simulink model "StarkQuadSimCL7772"  (R2018b)
settings: Solver=ode15s  StartTime=0.0  StopTime=Final_Time_1  RelTol=1e-3
values from neighbouring files (symbols this model uses):
  b = 1.0444e-4    (= 0.00010444)    [StarkQuad77.m]
  d = 7.3031e-6    (= 7.3031e-06)    [StarkQuad77.m]
  g = 9.81    [StarkQuad77.m]
  Index = int32(Index)    [StarkQuad77.m]
  Ixx = 5.296671410    (= 5.29667141)    [StarkQuad77.m]
  Iyy = 5.790964671    [StarkQuad77.m]
  Izz = 3.348512883    [StarkQuad77.m]
  l = 0.41123*2    (= 0.82246)    [StarkQuad77.m]
  M = [x z y]    [StarkQuad77.m]
  m = 10.800    (= 10.8)    [StarkQuad77.m]
  Psi_d = 10    [StarkQuad77.m]
  u1_max = b*4*speed_rads^2    (= 106.539244)    [StarkQuad77.m]
  u1_min = 0    [StarkQuad77.m]
  u2_max = b*l*speed_rads^2    (= 21.9060666551)    [StarkQuad77.m]
  u2_min = -u2_max    (= -21.9060666551)    [StarkQuad77.m]
  u3_max = u2_max    (= 21.9060666551)    [StarkQuad77.m]
  u3_min = u2_min    (= -21.9060666551)    [StarkQuad77.m]
  u4_max = d*l*2*speed_rads^2    (= 3.06361921464)    [StarkQuad77.m]
  u4_min = -u4_max    (= -3.06361921464)    [StarkQuad77.m]
  xp = CP.x(end)    [StarkQuad77.m]
  yp = CP.y(end)    [StarkQuad77.m]
libraries: simulink x6, powerlib_meascontrol x3, aerolibutil x2, vrlib x1
settings Model: Creator=cindyiskandar  LastModifiedBy=Anthony

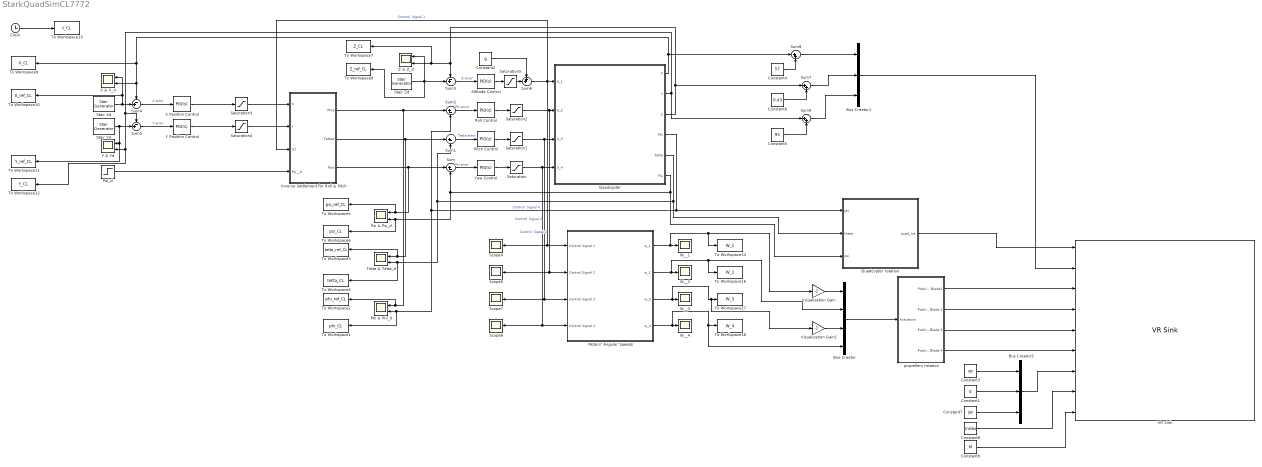
== system StarkQuadSimCL7772 ==
  "Altitude Control " : simulink/Continuous/PID Controller  Controller=PID  Form=Parallel  TimeDomain=Continuous-time  SampleTime=-1  IntegratorMethod=Forward Euler  FilterMethod=Forward Euler  ControllerParametersSource=internal  P=450  I=25  D=600  UseFilter=on  N=100  TunerSelectOption=Transfer Function Based (PID Tuner App)  InitialConditionSource=internal  InitialConditionForIntegrator=0  InitialConditionForFilter=0  DifferentiatorICPrevScaledInput=0  ExternalReset=none  TrackingMode=off  Kt=1  LimitOutput=off  UpperSaturationLimit=inf  LowerSaturationLimit=-inf  LinearizeAsGain=on  AntiWindupMode=none  Kb=1  POutMin=[]  POutMax=[]  IOutMin=[]  IOutMax=[]  DOutMin=[]  DOutMax=[]  NOutMin=[]  NOutMax=[]  SumOutMin=[]  SumOutMax=[]  SaturationOutMin=[]  SaturationOutMax=[]  PParamMin=[]  PParamMax=[]  IParamMin=[]  IParamMax=[]  DParamMin=[]  DParamMax=[]  NParamMin=[]  NParamMax=[]  KbParamMin=[]  KbParamMax=[]  KtParamMin=[]  KtParamMax=[]  KbOutMin=[]  KbOutMax=[]  KtOutMin=[]  KtOutMax=[]  IntegratorOutMin=[]  IntegratorOutMax=[]  FilterOutMin=[]  FilterOutMax=[]  SumI1OutMin=[]  SumI1OutMax=[]  SumI2OutMin=[]  SumI2OutMax=[]  SumI3OutMin=[]  SumI3OutMax=[]  SumI4OutMin=[]  SumI4OutMax=[]  SumDOutMin=[]  SumDOutMax=[]  DifferentiatorOutMin=[]  DifferentiatorOutMax=[]  FilterDiffOutCoefMin=[]  FilterDiffOutCoefMax=[]  ReciprocalOutMin=[]  ReciprocalOutMax=[]  SumDenOutMin=[]  SumDenOutMax=[]  SumNumOutMin=[]  SumNumOutMax=[]  DivideOutMin=[]  DivideOutMax=[]  IntegratorContinuousStateAttributes=''  IntegratorStateMustResolveToSignalObject=off  IntegratorRTWStateStorageClass=Auto  FilterContinuousStateAttributes=''  FilterStateMustResolveToSignalObject=off  FilterRTWStateStorageClass=Auto  ParallelPVariant=InternalParameters  IdealPVariant=Disabled  IVariant=InternalParameters  DVariant=InternalParameters  IntegratorVariant=Continuous  SatVariant=Disabled  AWVariant=Passthrough  PCopyVariant=Disabled  TRVariant=Disabled  FdbkBlocksVariant=Forward  IdealPFdbkVariant=Disabled  SatFdbkVariant=Disabled  DerivativeFilterVariant=ContFilter  NVariant=InternalParameters  NCopyVariant=Disabled  FilterICVariant=InternalICsFilter  IntegratorICVariant=InternalICs  ExternalResetVariant=Disabled  TRSumVariant=Passthrough  SumFdbkVariant=Disabled  SumVariant=Sum_PID
  Bus Creator : BusCreator  Inputs=4
  Bus Creator1 : BusCreator  Inputs=3
  Bus Creator2 : BusCreator  Inputs=3
  Clock : Clock
  Constant1 : Constant  Value=0
  Constant2 : Constant  Value=g
  Constant3 : Constant  Value=xp
  Constant4 : Constant  Value=57
  Constant5 : Constant  Value=95
  Constant6 : Constant  Value=0.43
  Constant7 : Constant  Value=yp
  Constant8 : Constant  Value=Index  VectorParams1D=off
  Constant9 : Constant  Value=M
  Inverse Settlement for Roll & Pitch : Subsystem
  Motors' Angular Speeds : Subsystem
  "Phi & Phi_d " : Scope  NumInputPorts=2
  Pitch Control : simulink/Continuous/PID Controller  Controller=PID  Form=Parallel  TimeDomain=Continuous-time  SampleTime=-1  IntegratorMethod=Forward Euler  FilterMethod=Forward Euler  ControllerParametersSource=internal  P=226  I=0  D=320  UseFilter=on  N=100  TunerSelectOption=Transfer Function Based (PID Tuner App)  InitialConditionSource=internal  InitialConditionForIntegrator=0  InitialConditionForFilter=0  DifferentiatorICPrevScaledInput=0  ExternalReset=none  TrackingMode=off  Kt=1  LimitOutput=off  UpperSaturationLimit=inf  LowerSaturationLimit=-inf  LinearizeAsGain=on  AntiWindupMode=none  Kb=1  POutMin=[]  POutMax=[]  IOutMin=[]  IOutMax=[]  DOutMin=[]  DOutMax=[]  NOutMin=[]  NOutMax=[]  SumOutMin=[]  SumOutMax=[]  SaturationOutMin=[]  SaturationOutMax=[]  PParamMin=[]  PParamMax=[]  IParamMin=[]  IParamMax=[]  DParamMin=[]  DParamMax=[]  NParamMin=[]  NParamMax=[]  KbParamMin=[]  KbParamMax=[]  KtParamMin=[]  KtParamMax=[]  KbOutMin=[]  KbOutMax=[]  KtOutMin=[]  KtOutMax=[]  IntegratorOutMin=[]  IntegratorOutMax=[]  FilterOutMin=[]  FilterOutMax=[]  SumI1OutMin=[]  SumI1OutMax=[]  SumI2OutMin=[]  SumI2OutMax=[]  SumI3OutMin=[]  SumI3OutMax=[]  SumI4OutMin=[]  SumI4OutMax=[]  SumDOutMin=[]  SumDOutMax=[]  DifferentiatorOutMin=[]  DifferentiatorOutMax=[]  FilterDiffOutCoefMin=[]  FilterDiffOutCoefMax=[]  ReciprocalOutMin=[]  ReciprocalOutMax=[]  SumDenOutMin=[]  SumDenOutMax=[]  SumNumOutMin=[]  SumNumOutMax=[]  DivideOutMin=[]  DivideOutMax=[]  IntegratorContinuousStateAttributes=''  IntegratorStateMustResolveToSignalObject=off  IntegratorRTWStateStorageClass=Auto  FilterContinuousStateAttributes=''  FilterStateMustResolveToSignalObject=off  FilterRTWStateStorageClass=Auto  ParallelPVariant=InternalParameters  IdealPVariant=Disabled  IVariant=InternalParameters  DVariant=InternalParameters  IntegratorVariant=Continuous  SatVariant=Disabled  AWVariant=Passthrough  PCopyVariant=Disabled  TRVariant=Disabled  FdbkBlocksVariant=Forward  IdealPFdbkVariant=Disabled  SatFdbkVariant=Disabled  DerivativeFilterVariant=ContFilter  NVariant=InternalParameters  NCopyVariant=Disabled  FilterICVariant=InternalICsFilter  IntegratorICVariant=InternalICs  ExternalResetVariant=Disabled  TRSumVariant=Passthrough  SumFdbkVariant=Disabled  SumVariant=Sum_PID
  Psi & Psi_d : Scope  NumInputPorts=2
  Psi_d : Step  After=Psi_d  SampleTime=0
  Quadcopter : Subsystem
  Quadcopter rotation : Subsystem
  Roll Control : simulink/Continuous/PID Controller  Controller=PID  Form=Parallel  TimeDomain=Continuous-time  SampleTime=-1  IntegratorMethod=Forward Euler  FilterMethod=Forward Euler  ControllerParametersSource=internal  P=290  I=0  D=320  UseFilter=on  N=100  TunerSelectOption=Transfer Function Based (PID Tuner App)  InitialConditionSource=internal  InitialConditionForIntegrator=0  InitialConditionForFilter=0  DifferentiatorICPrevScaledInput=0  ExternalReset=none  TrackingMode=off  Kt=1  LimitOutput=off  UpperSaturationLimit=inf  LowerSaturationLimit=-inf  LinearizeAsGain=on  AntiWindupMode=none  Kb=1  POutMin=[]  POutMax=[]  IOutMin=[]  IOutMax=[]  DOutMin=[]  DOutMax=[]  NOutMin=[]  NOutMax=[]  SumOutMin=[]  SumOutMax=[]  SaturationOutMin=[]  SaturationOutMax=[]  PParamMin=[]  PParamMax=[]  IParamMin=[]  IParamMax=[]  DParamMin=[]  DParamMax=[]  NParamMin=[]  NParamMax=[]  KbParamMin=[]  KbParamMax=[]  KtParamMin=[]  KtParamMax=[]  KbOutMin=[]  KbOutMax=[]  KtOutMin=[]  KtOutMax=[]  IntegratorOutMin=[]  IntegratorOutMax=[]  FilterOutMin=[]  FilterOutMax=[]  SumI1OutMin=[]  SumI1OutMax=[]  SumI2OutMin=[]  SumI2OutMax=[]  SumI3OutMin=[]  SumI3OutMax=[]  SumI4OutMin=[]  SumI4OutMax=[]  SumDOutMin=[]  SumDOutMax=[]  DifferentiatorOutMin=[]  DifferentiatorOutMax=[]  FilterDiffOutCoefMin=[]  FilterDiffOutCoefMax=[]  ReciprocalOutMin=[]  ReciprocalOutMax=[]  SumDenOutMin=[]  SumDenOutMax=[]  SumNumOutMin=[]  SumNumOutMax=[]  DivideOutMin=[]  DivideOutMax=[]  IntegratorContinuousStateAttributes=''  IntegratorStateMustResolveToSignalObject=off  IntegratorRTWStateStorageClass=Auto  FilterContinuousStateAttributes=''  FilterStateMustResolveToSignalObject=off  FilterRTWStateStorageClass=Auto  ParallelPVariant=InternalParameters  IdealPVariant=Disabled  IVariant=InternalParameters  DVariant=InternalParameters  IntegratorVariant=Continuous  SatVariant=Disabled  AWVariant=Passthrough  PCopyVariant=Disabled  TRVariant=Disabled  FdbkBlocksVariant=Forward  IdealPFdbkVariant=Disabled  SatFdbkVariant=Disabled  DerivativeFilterVariant=ContFilter  NVariant=InternalParameters  NCopyVariant=Disabled  FilterICVariant=InternalICsFilter  IntegratorICVariant=InternalICs  ExternalResetVariant=Disabled  TRSumVariant=Passthrough  SumFdbkVariant=Disabled  SumVariant=Sum_PID
  Saturation : Saturate  UpperLimit=u4_max  LowerLimit=u4_min
  Saturation1 : Saturate  UpperLimit=u3_max  LowerLimit=u3_min
  Saturation2 : Saturate  UpperLimit=u2_max  LowerLimit=u2_min
  Saturation3 : Saturate  UpperLimit=3*g  LowerLimit=-3*g
  Saturation4 : Saturate  UpperLimit=3*g  LowerLimit=-3*g
  Saturation5 : Saturate  UpperLimit=u1_max  LowerLimit=u1_min
  Scope{4..7} (4 alike) : Scope
  Stair Xd : powerlib_meascontrol/Pulse & Signal Generators/Stair Generator  t=Time  e=Xd  Ts=0
      settings: SourceProductName=Simscape Power Systems
  Stair Yd : powerlib_meascontrol/Pulse & Signal Generators/Stair Generator  t=Time  e=Yd  Ts=0
      settings: SourceProductName=Simscape Power Systems
  Stair Zd : powerlib_meascontrol/Pulse & Signal Generators/Stair Generator  t=Time  e=Zd  Ts=0
      settings: SourceProductName=Simscape Power Systems
  Sum : Sum  Inputs=|+-
  Sum1 : Sum  Inputs=|+-
  Sum2 : Sum  Inputs=|+-
  Sum3 : Sum  Inputs=-+|
  Sum4 : Sum  Inputs=-+|
  Sum5 : Sum  Inputs=-+|
  Sum6 : Sum  Inputs=++|
  Sum7 : Sum  Inputs=|++
  Sum8 : Sum  Inputs=|++
  Sum9 : Sum  Inputs=|++
  "Tetta & Tetta_d " : Scope  NumInputPorts=2
  To Workspace1 : ToWorkspace  VariableName=phi_CL  SampleTime=-1
      settings: Save2DSignal=2-D array (concatenate along first dimension)
  To Workspace10 : ToWorkspace  VariableName=X_ref_CL  SampleTime=-1
      settings: Save2DSignal=2-D array (concatenate along first dimension)
  To Workspace11 : ToWorkspace  VariableName=Y_ref_CL  SampleTime=-1
      settings: Save2DSignal=2-D array (concatenate along first dimension)
  To Workspace12 : ToWorkspace  VariableName=Y_CL  SampleTime=-1
      settings: Save2DSignal=2-D array (concatenate along first dimension)
  To Workspace13 : ToWorkspace  VariableName=t_CL  SampleTime=-1
      settings: Save2DSignal=2-D array (concatenate along first dimension)
  To Workspace14 : ToWorkspace  VariableName=W_1  SampleTime=-1
      settings: Save2DSignal=2-D array (concatenate along first dimension)
  To Workspace16 : ToWorkspace  VariableName=W_2  SampleTime=-1
      settings: Save2DSignal=2-D array (concatenate along first dimension)
  To Workspace17 : ToWorkspace  VariableName=W_3  SampleTime=-1
      settings: Save2DSignal=2-D array (concatenate along first dimension)
  To Workspace18 : ToWorkspace  VariableName=W_4  SampleTime=-1
      settings: Save2DSignal=2-D array (concatenate along first dimension)
  To Workspace2 : ToWorkspace  VariableName=phi_ref_CL  SampleTime=-1
      settings: Save2DSignal=2-D array (concatenate along first dimension)
  To Workspace3 : ToWorkspace  VariableName=tetta_ref_CL  SampleTime=-1
      settings: Save2DSignal=2-D array (concatenate along first dimension)
  To Workspace4 : ToWorkspace  VariableName=tetta_CL  SampleTime=-1
      settings: Save2DSignal=2-D array (concatenate along first dimension)
  To Workspace5 : ToWorkspace  VariableName=psi_ref_CL  SampleTime=-1
      settings: Save2DSignal=2-D array (concatenate along first dimension)
  To Workspace6 : ToWorkspace  VariableName=psi_CL  SampleTime=-1
      settings: Save2DSignal=2-D array (concatenate along first dimension)
  To Workspace7 : ToWorkspace  VariableName=Z_CL  SampleTime=-1
      settings: Save2DSignal=2-D array (concatenate along first dimension)
  To Workspace8 : ToWorkspace  VariableName=Z_ref_CL  SampleTime=-1
      settings: Save2DSignal=2-D array (concatenate along first dimension)
  To Workspace9 : ToWorkspace  VariableName=X_CL  SampleTime=-1
      settings: Save2DSignal=2-D array (concatenate along first dimension)
  VR Sink : vrlib/VR Sink  InstantiateOnLoad=on  SampleTime=0.1  ViewEnable=on  RemoteChange=off  RemoteView=off  FieldsWritten=quadcopter.rotation.4.1.1.double#quadcopter.translation.3.1.1.double#blade1.rotation.4.1.1.double#blade2.rotation.4.1.1.double#blade3.rotation.4.1.1.double#blade4.rotation.4.1.1.double#LandingMarker_Waypoint.translation.3.1.1.double#LineIndexedList.coordIndex.1.-1.1.double#LineCoordinates.point.3.-1.1.double  WorldFileName=VR.wrl  AutoView=on  VideoDimensions=[]  AllowVariableSize=off  FigureProperties="{'Position', 'Name', 'Viewpoint', 'CameraBound', 'CameraDirection', 'CameraPosition', 'CameraUpVector', 'ZoomFactor', 'Antialiasing', 'Headlight', 'Lighting', 'NavPanel', 'Sound', 'StatusBar', 'Stereo3D', 'Stereo3DCameraOffset', 'Stereo3DHIT', 'ToolBar', 'Textures', 'Transparency', 'Triad', 'Wireframe', 'NavZones', 'NavMode', 'NavSpeed', 'CaptureFileFormat', 'CaptureFileName', 'Record2DCompressMethod', 'Record2DCompressQuality', 'Record2D', 'Record2DFileName', 'Record2DFPS'; [1.0000000000000000e+00   7.4199999999999932e+01   1.5360000000000000e+03   6.9880000000000007e+02], '', 'Isometric', 'on', [0.0000000000000000e+00   0.0000000000000000e+00  -1.0000000000000000e+00], [0.0000000000000000e+00   0.0000000000000000e+00   0.0000000000000000e+00], [0.0000000000000000e+00   1.0000000000000000e+00   0.0000000000000000e+00], [1.0000000000000000e+00], 'on', 'on', 'on', 'halfbar', 'on', 'on', 'off', [1.0000000149011612e-01], [0.0000000000000000e+00], 'on', 'on', 'on', 'none', 'off', 'off', 'fly', 'normal', 'tif', '%f_anim_%n.tif', 'auto', [7.5000000000000000e+01], 'off', '%f_anim_%n.avi', 'auto'}"
      settings: SourceProductBaseCode=VR
  Visualization Gain : Gain  Gain=-1
  Visualization Gain1 : Gain  Gain=-1
  W__{1..4} (4 alike) : Scope
  X & X_d : Scope  NumInputPorts=2
  X Position Control : simulink/Continuous/PID Controller  Controller=PID  Form=Parallel  TimeDomain=Continuous-time  SampleTime=-1  IntegratorMethod=Forward Euler  FilterMethod=Forward Euler  ControllerParametersSource=internal  P=0.7  I=0  D=5  UseFilter=on  N=100  TunerSelectOption=Transfer Function Based (PID Tuner App)  InitialConditionSource=internal  InitialConditionForIntegrator=0  InitialConditionForFilter=0  DifferentiatorICPrevScaledInput=0  ExternalReset=none  TrackingMode=off  Kt=1  LimitOutput=off  UpperSaturationLimit=inf  LowerSaturationLimit=-inf  LinearizeAsGain=on  AntiWindupMode=none  Kb=1  POutMin=[]  POutMax=[]  IOutMin=[]  IOutMax=[]  DOutMin=[]  DOutMax=[]  NOutMin=[]  NOutMax=[]  SumOutMin=[]  SumOutMax=[]  SaturationOutMin=[]  SaturationOutMax=[]  PParamMin=[]  PParamMax=[]  IParamMin=[]  IParamMax=[]  DParamMin=[]  DParamMax=[]  NParamMin=[]  NParamMax=[]  KbParamMin=[]  KbParamMax=[]  KtParamMin=[]  KtParamMax=[]  KbOutMin=[]  KbOutMax=[]  KtOutMin=[]  KtOutMax=[]  IntegratorOutMin=[]  IntegratorOutMax=[]  FilterOutMin=[]  FilterOutMax=[]  SumI1OutMin=[]  SumI1OutMax=[]  SumI2OutMin=[]  SumI2OutMax=[]  SumI3OutMin=[]  SumI3OutMax=[]  SumI4OutMin=[]  SumI4OutMax=[]  SumDOutMin=[]  SumDOutMax=[]  DifferentiatorOutMin=[]  DifferentiatorOutMax=[]  FilterDiffOutCoefMin=[]  FilterDiffOutCoefMax=[]  ReciprocalOutMin=[]  ReciprocalOutMax=[]  SumDenOutMin=[]  SumDenOutMax=[]  SumNumOutMin=[]  SumNumOutMax=[]  DivideOutMin=[]  DivideOutMax=[]  IntegratorContinuousStateAttributes=''  IntegratorStateMustResolveToSignalObject=off  IntegratorRTWStateStorageClass=Auto  FilterContinuousStateAttributes=''  FilterStateMustResolveToSignalObject=off  FilterRTWStateStorageClass=Auto  ParallelPVariant=InternalParameters  IdealPVariant=Disabled  IVariant=InternalParameters  DVariant=InternalParameters  IntegratorVariant=Continuous  SatVariant=Disabled  AWVariant=Passthrough  PCopyVariant=Disabled  TRVariant=Disabled  FdbkBlocksVariant=Forward  IdealPFdbkVariant=Disabled  SatFdbkVariant=Disabled  DerivativeFilterVariant=ContFilter  NVariant=InternalParameters  NCopyVariant=Disabled  FilterICVariant=InternalICsFilter  IntegratorICVariant=InternalICs  ExternalResetVariant=Disabled  TRSumVariant=Passthrough  SumFdbkVariant=Disabled  SumVariant=Sum_PID
  Y & Yd : Scope  NumInputPorts=2
  Y Position Control : simulink/Continuous/PID Controller  Controller=PID  Form=Parallel  TimeDomain=Continuous-time  SampleTime=-1  IntegratorMethod=Forward Euler  FilterMethod=Forward Euler  ControllerParametersSource=internal  P=0.7  I=0  D=5  UseFilter=on  N=100  TunerSelectOption=Transfer Function Based (PID Tuner App)  InitialConditionSource=internal  InitialConditionForIntegrator=0  InitialConditionForFilter=0  DifferentiatorICPrevScaledInput=0  ExternalReset=none  TrackingMode=off  Kt=1  LimitOutput=off  UpperSaturationLimit=inf  LowerSaturationLimit=-inf  LinearizeAsGain=on  AntiWindupMode=none  Kb=1  POutMin=[]  POutMax=[]  IOutMin=[]  IOutMax=[]  DOutMin=[]  DOutMax=[]  NOutMin=[]  NOutMax=[]  SumOutMin=[]  SumOutMax=[]  SaturationOutMin=[]  SaturationOutMax=[]  PParamMin=[]  PParamMax=[]  IParamMin=[]  IParamMax=[]  DParamMin=[]  DParamMax=[]  NParamMin=[]  NParamMax=[]  KbParamMin=[]  KbParamMax=[]  KtParamMin=[]  KtParamMax=[]  KbOutMin=[]  KbOutMax=[]  KtOutMin=[]  KtOutMax=[]  IntegratorOutMin=[]  IntegratorOutMax=[]  FilterOutMin=[]  FilterOutMax=[]  SumI1OutMin=[]  SumI1OutMax=[]  SumI2OutMin=[]  SumI2OutMax=[]  SumI3OutMin=[]  SumI3OutMax=[]  SumI4OutMin=[]  SumI4OutMax=[]  SumDOutMin=[]  SumDOutMax=[]  DifferentiatorOutMin=[]  DifferentiatorOutMax=[]  FilterDiffOutCoefMin=[]  FilterDiffOutCoefMax=[]  ReciprocalOutMin=[]  ReciprocalOutMax=[]  SumDenOutMin=[]  SumDenOutMax=[]  SumNumOutMin=[]  SumNumOutMax=[]  DivideOutMin=[]  DivideOutMax=[]  IntegratorContinuousStateAttributes=''  IntegratorStateMustResolveToSignalObject=off  IntegratorRTWStateStorageClass=Auto  FilterContinuousStateAttributes=''  FilterStateMustResolveToSignalObject=off  FilterRTWStateStorageClass=Auto  ParallelPVariant=InternalParameters  IdealPVariant=Disabled  IVariant=InternalParameters  DVariant=InternalParameters  IntegratorVariant=Continuous  SatVariant=Disabled  AWVariant=Passthrough  PCopyVariant=Disabled  TRVariant=Disabled  FdbkBlocksVariant=Forward  IdealPFdbkVariant=Disabled  SatFdbkVariant=Disabled  DerivativeFilterVariant=ContFilter  NVariant=InternalParameters  NCopyVariant=Disabled  FilterICVariant=InternalICsFilter  IntegratorICVariant=InternalICs  ExternalResetVariant=Disabled  TRSumVariant=Passthrough  SumFdbkVariant=Disabled  SumVariant=Sum_PID
  Yaw Control : simulink/Continuous/PID Controller  Controller=PID  Form=Parallel  TimeDomain=Continuous-time  SampleTime=-1  IntegratorMethod=Forward Euler  FilterMethod=Forward Euler  ControllerParametersSource=internal  P=193  I=0  D=320  UseFilter=on  N=100  TunerSelectOption=Transfer Function Based (PID Tuner App)  InitialConditionSource=internal  InitialConditionForIntegrator=0  InitialConditionForFilter=0  DifferentiatorICPrevScaledInput=0  ExternalReset=none  TrackingMode=off  Kt=1  LimitOutput=off  UpperSaturationLimit=inf  LowerSaturationLimit=-inf  LinearizeAsGain=on  AntiWindupMode=none  Kb=1  POutMin=[]  POutMax=[]  IOutMin=[]  IOutMax=[]  DOutMin=[]  DOutMax=[]  NOutMin=[]  NOutMax=[]  SumOutMin=[]  SumOutMax=[]  SaturationOutMin=[]  SaturationOutMax=[]  PParamMin=[]  PParamMax=[]  IParamMin=[]  IParamMax=[]  DParamMin=[]  DParamMax=[]  NParamMin=[]  NParamMax=[]  KbParamMin=[]  KbParamMax=[]  KtParamMin=[]  KtParamMax=[]  KbOutMin=[]  KbOutMax=[]  KtOutMin=[]  KtOutMax=[]  IntegratorOutMin=[]  IntegratorOutMax=[]  FilterOutMin=[]  FilterOutMax=[]  SumI1OutMin=[]  SumI1OutMax=[]  SumI2OutMin=[]  SumI2OutMax=[]  SumI3OutMin=[]  SumI3OutMax=[]  SumI4OutMin=[]  SumI4OutMax=[]  SumDOutMin=[]  SumDOutMax=[]  DifferentiatorOutMin=[]  DifferentiatorOutMax=[]  FilterDiffOutCoefMin=[]  FilterDiffOutCoefMax=[]  ReciprocalOutMin=[]  ReciprocalOutMax=[]  SumDenOutMin=[]  SumDenOutMax=[]  SumNumOutMin=[]  SumNumOutMax=[]  DivideOutMin=[]  DivideOutMax=[]  IntegratorContinuousStateAttributes=''  IntegratorStateMustResolveToSignalObject=off  IntegratorRTWStateStorageClass=Auto  FilterContinuousStateAttributes=''  FilterStateMustResolveToSignalObject=off  FilterRTWStateStorageClass=Auto  ParallelPVariant=InternalParameters  IdealPVariant=Disabled  IVariant=InternalParameters  DVariant=InternalParameters  IntegratorVariant=Continuous  SatVariant=Disabled  AWVariant=Passthrough  PCopyVariant=Disabled  TRVariant=Disabled  FdbkBlocksVariant=Forward  IdealPFdbkVariant=Disabled  SatFdbkVariant=Disabled  DerivativeFilterVariant=ContFilter  NVariant=InternalParameters  NCopyVariant=Disabled  FilterICVariant=InternalICsFilter  IntegratorICVariant=InternalICs  ExternalResetVariant=Disabled  TRSumVariant=Passthrough  SumFdbkVariant=Disabled  SumVariant=Sum_PID
  Z & Z_d : Scope  NumInputPorts=2
  propellers rotation : Subsystem
  wires:
  Sum/1 -> Yaw Control/1  "Psi error"
  Sum1/1 -> Pitch Control/1  "Tetta error"
  Sum2/1 -> Roll Control/1  "Phi error"
  Sum4/1 -> X Position Control/1  "X error"
  Sum5/1 -> Y Position Control/1  "Y error"
  Yaw Control/1 -> Saturation/1
  Pitch Control/1 -> Saturation1/1
  Roll Control/1 -> Saturation2/1
  Sum3/1 -> "Altitude Control "/1  "Z error"
  X Position Control/1 -> Saturation3/1
  Y Position Control/1 -> Saturation4/1
  Saturation3/1 -> Inverse Settlement for Roll & Pitch/1(X)
  Saturation4/1 -> Inverse Settlement for Roll & Pitch/2(Y)
  Psi_d/1 -> Inverse Settlement for Roll & Pitch/4(Psi__d)
  Inverse Settlement for Roll & Pitch/1("Phid ") -> Sum2/1, To Workspace2/1, "Phi & Phi_d "/1
  Inverse Settlement for Roll & Pitch/2(Tettad) -> Sum1/1, To Workspace3/1, "Tetta & Tetta_d "/1
  Inverse Settlement for Roll & Pitch/3("Psid ") -> To Workspace5/1, Psi & Psi_d/1, Sum/1
  Stair Zd/1 -> To Workspace8/1, Z & Z_d/1, Sum3/2
  Stair Xd/1 -> X & X_d/1, To Workspace10/1, Sum4/2
  Stair Yd/1 -> To Workspace11/1, Y & Yd/1, Sum5/2
  Clock/1 -> To Workspace13/1
  Saturation/1 -> Quadcopter/4(U_4), Scope6/1, Motors' Angular Speeds/4(Control Signal 4)  "Control  Signal 4"
  "Altitude Control "/1 -> Saturation5/1
  Saturation2/1 -> Motors' Angular Speeds/2(Control Signal 2), Scope5/1, Quadcopter/2(U_2)  "Control  Signal 2"
  Saturation1/1 -> Quadcopter/3(U_3), Motors' Angular Speeds/3(Control Signal 3), Scope7/1  "Control  Signal 3"
  Constant2/1 -> Sum6/1
  Sum6/1 -> Inverse Settlement for Roll & Pitch/3(U1), Motors' Angular Speeds/1(Control Signal 1), Scope4/1, Quadcopter/1(U_1)  "Control  Signal 1"
  Saturation5/1 -> Sum6/2
  Sum7/1 -> Bus Creator1/2
  Quadcopter/3(Z) -> To Workspace7/1, Z & Z_d/2, Sum3/1, Sum7/1
  Motors' Angular Speeds/1(w_1) -> Visualization Gain/1, To Workspace14/1, W__1/1
  Motors' Angular Speeds/4(w_4) -> To Workspace18/1, Bus Creator/4, W__4/1
  Constant4/1 -> Sum8/2
  Constant6/1 -> Sum7/2
  Motors' Angular Speeds/2(w_2) -> Bus Creator/2, To Workspace16/1, W__2/1
  Constant5/1 -> Sum9/2
  Visualization Gain/1 -> Bus Creator/1
  Visualization Gain1/1 -> Bus Creator/3
  Bus Creator/1 -> propellers rotation/1(Actuators)
  Motors' Angular Speeds/3(w_3) -> Visualization Gain1/1, To Workspace17/1, W__3/1
  Quadcopter/1(X) -> Sum4/1, X & X_d/2, To Workspace9/1, Sum8/1
  Quadcopter/6(Psi) -> Quadcopter rotation/3(psi), To Workspace6/1, Psi & Psi_d/2, Sum/2
  Sum9/1 -> Bus Creator1/3
  Sum8/1 -> Bus Creator1/1
  Quadcopter/4(Phi) -> Quadcopter rotation/1(phi), To Workspace1/1, "Phi & Phi_d "/2, Sum2/2
  Quadcopter/2(Y) -> Sum9/1, To Workspace12/1, Y & Yd/2, Sum5/1
  Quadcopter/5(Tetta) -> Quadcopter rotation/2(theta), To Workspace4/1, "Tetta & Tetta_d "/2, Sum1/2
  Constant3/1 -> Bus Creator2/1
  Constant1/1 -> Bus Creator2/2
  Constant7/1 -> Bus Creator2/3
  Constant9/1 -> VR Sink/9
  Constant8/1 -> VR Sink/8
  Bus Creator2/1 -> VR Sink/7
  propellers rotation/4(Position Blade 4) -> VR Sink/6
  propellers rotation/3(Position Blade 3) -> VR Sink/5
  propellers rotation/2(Position Blade 2) -> VR Sink/4
  propellers rotation/1(Position Blade1) -> VR Sink/3
  Quadcopter rotation/1(quad_rot) -> VR Sink/1
  Bus Creator1/1 -> VR Sink/2

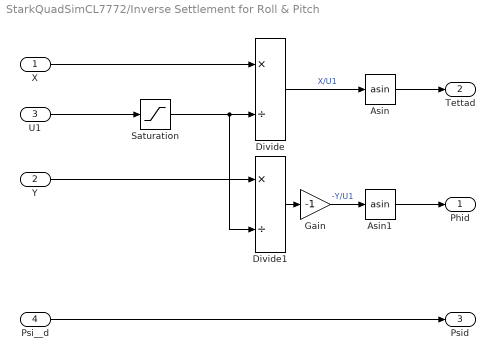
== system StarkQuadSimCL7772/Inverse Settlement for Roll & Pitch ==
  X : Inport
  Y : Inport  Port=2
  U1 : Inport  Port=3
  Psi__d : Inport  Port=4
  Asin : Trigonometry  Operator=asin
  Asin1 : Trigonometry  Operator=asin
  Divide : Product  Inputs=*/
  Divide1 : Product  Inputs=*/
  Gain : Gain  Gain=-1
  Saturation : Saturate  UpperLimit=u1_max  LowerLimit=0.01  OutMin=[0.01]  OutMax=[u1_max]
  "Phid " : Outport
  Tettad : Outport  Port=2
  "Psid " : Outport  Port=3
  wires:
  Asin1/1 -> "Phid "/1
  Gain/1 -> Asin1/1  "-Y/U1"
  Divide/1 -> Asin/1  "X/U1"
  U1/1 -> Saturation/1
  Divide1/1 -> Gain/1
  Asin/1 -> Tettad/1
  Psi__d/1 -> "Psid "/1
  Saturation/1 -> Divide1/2, Divide/2
  X/1 -> Divide/1
  Y/1 -> Divide1/1

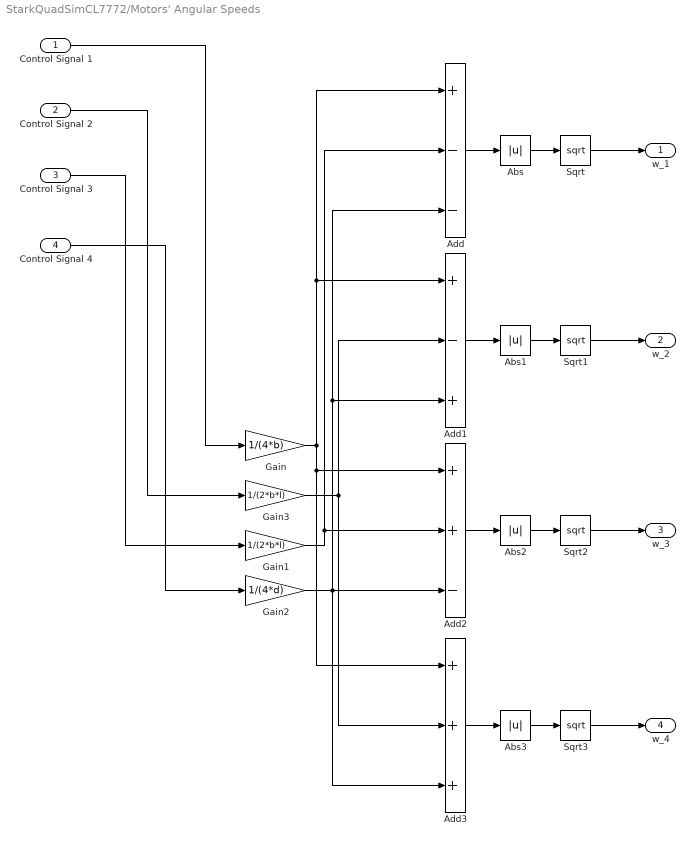
== system StarkQuadSimCL7772/Motors' Angular Speeds ==
  Control Signal 1 : Inport
  Control Signal 2 : Inport  Port=2
  Control Signal 3 : Inport  Port=3
  Control Signal 4 : Inport  Port=4
  Abs{,1..3} (4 alike) : Abs
  Add : Sum  Inputs=+--
  Add1 : Sum  Inputs=+-+
  Add2 : Sum  Inputs=++-
  Add3 : Sum  Inputs=+++
  Gain : Gain  Gain=1/(4*b)
  Gain1 : Gain  Gain=1/(2*b*l)
  Gain2 : Gain  Gain=1/(4*d)
  Gain3 : Gain  Gain=1/(2*b*l)
  Sqrt{,1..3} (4 alike) : Sqrt  SaturateOnIntegerOverflow=on
  w_1 : Outport
  w_2 : Outport  Port=2
  w_3 : Outport  Port=3
  w_4 : Outport  Port=4
  wires:
  Control Signal 1/1 -> Gain/1
  Control Signal 3/1 -> Gain1/1
  Sqrt2/1 -> w_3/1
  Sqrt3/1 -> w_4/1
  Control Signal 4/1 -> Gain2/1
  Sqrt/1 -> w_1/1
  Gain2/1 -> Add1/3, Add/3, Add3/3, Add2/3
  Gain1/1 -> Add/2, Add2/2
  Sqrt1/1 -> w_2/1
  Gain/1 -> Add1/1, Add/1, Add3/1, Add2/1
  Control Signal 2/1 -> Gain3/1
  Gain3/1 -> Add3/2, Add1/2
  Add/1 -> Abs/1
  Add3/1 -> Abs3/1
  Add2/1 -> Abs2/1
  Add1/1 -> Abs1/1
  Abs/1 -> Sqrt/1
  Abs3/1 -> Sqrt3/1
  Abs2/1 -> Sqrt2/1
  Abs1/1 -> Sqrt1/1

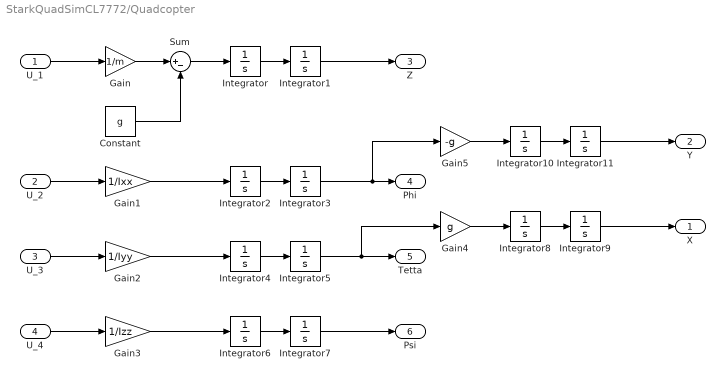
== system StarkQuadSimCL7772/Quadcopter ==
  U_1 : Inport
  U_2 : Inport  Port=2
  U_3 : Inport  Port=3
  U_4 : Inport  Port=4
  Constant : Constant  Value=g
  Gain : Gain  Gain=1/m
  Gain1 : Gain  Gain=1/Ixx
  Gain2 : Gain  Gain=1/Iyy
  Gain3 : Gain  Gain=1/Izz
  Gain4 : Gain  Gain=g
  Gain5 : Gain  Gain=-g
  Integrator{,1..11} (12 alike) : Integrator
  Sum : Sum  Inputs=|+-
  X : Outport
  Y : Outport  Port=2
  Z : Outport  Port=3
  Phi : Outport  Port=4
  Tetta : Outport  Port=5
  Psi : Outport  Port=6
  wires:
  Integrator4/1 -> Integrator5/1
  Gain3/1 -> Integrator6/1
  U_3/1 -> Gain2/1
  Integrator5/1 -> Tetta/1, Gain4/1
  U_4/1 -> Gain3/1
  Gain2/1 -> Integrator4/1
  Gain1/1 -> Integrator2/1
  Integrator6/1 -> Integrator7/1
  Integrator7/1 -> Psi/1
  U_1/1 -> Gain/1
  U_2/1 -> Gain1/1
  Gain/1 -> Sum/1
  Sum/1 -> Integrator/1
  Integrator2/1 -> Integrator3/1
  Integrator3/1 -> Gain5/1, Phi/1
  Integrator1/1 -> Z/1
  Gain4/1 -> Integrator8/1
  Integrator/1 -> Integrator1/1
  Integrator9/1 -> X/1
  Integrator8/1 -> Integrator9/1
  Constant/1 -> Sum/2
  Integrator10/1 -> Integrator11/1
  Integrator11/1 -> Y/1
  Gain5/1 -> Integrator10/1

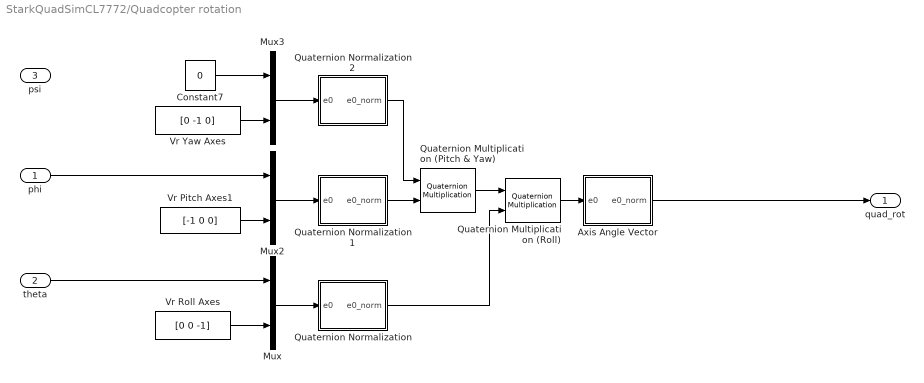
== system StarkQuadSimCL7772/Quadcopter rotation ==
  phi : Inport
  theta : Inport  Port=2
  psi : Inport  Port=3
  Axis Angle Vector : Subsystem
  Constant7 : Constant  Value=0
  Mux : Mux  Inputs=2
  Mux2 : Mux  Inputs=2
  Mux3 : Mux  Inputs=2
  Quaternion Multiplication (Pitch & Yaw) : aerolibutil/Quaternion Multiplication
  Quaternion Multiplication (Roll) : aerolibutil/Quaternion Multiplication
  Quaternion Normalization : Subsystem
  Quaternion Normalization1 : Subsystem
  Quaternion Normalization2 : Subsystem
  Vr Pitch Axes1 : Constant  Value=[-1 0 0]
  Vr Roll Axes : Constant  Value=[0 0 -1]
  Vr Yaw Axes : Constant  Value=[0 -1 0]
  quad_rot : Outport
  wires:
  Vr Yaw Axes/1 -> Mux3/2
  Mux/1 -> Quaternion Normalization/1(e0)
  Quaternion Normalization/1(e0_norm) -> Quaternion Multiplication (Roll)/2
  Quaternion Normalization2/1(e0_norm) -> Quaternion Multiplication (Pitch & Yaw)/1
  Quaternion Normalization1/1(e0_norm) -> Quaternion Multiplication (Pitch & Yaw)/2
  Vr Pitch Axes1/1 -> Mux2/2
  Mux2/1 -> Quaternion Normalization1/1(e0)
  Quaternion Multiplication (Pitch & Yaw)/1 -> Quaternion Multiplication (Roll)/1
  Mux3/1 -> Quaternion Normalization2/1(e0)
  Vr Roll Axes/1 -> Mux/2
  Quaternion Multiplication (Roll)/1 -> Axis Angle Vector/1(e0)
  Constant7/1 -> Mux3/1
  theta/1 -> Mux/1
  phi/1 -> Mux2/1
  Axis Angle Vector/1(e0_norm) -> quad_rot/1

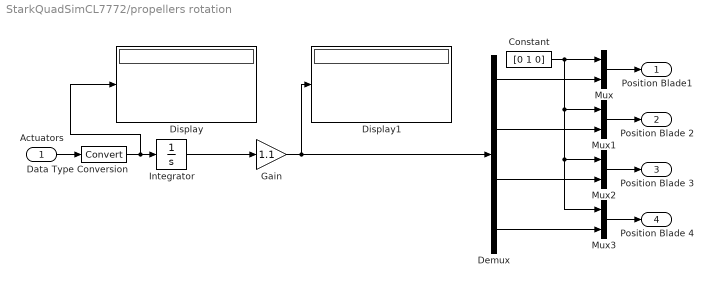
== system StarkQuadSimCL7772/propellers rotation ==
  Actuators : Inport
  Constant : Constant  Value=[0 1 0]
  Data Type Conversion : DataTypeConversion
  Demux : Demux
  Display : Display
  Display1 : Display
  Gain : Gain  Gain=1.1
  Integrator : Integrator  InitialCondition=[0 0 0 0]  WrappedStateUpperValue=2*pi  WrappedStateLowerValue=0
  Mux{,1..3} (4 alike) : Mux  Inputs=2
  Position Blade1 : Outport
  Position Blade 2 : Outport  Port=2
  Position Blade 3 : Outport  Port=3
  Position Blade 4 : Outport  Port=4
  wires:
  Demux/4 -> Mux3/2
  Mux3/1 -> Position Blade 4/1
  Demux/2 -> Mux1/2
  Demux/3 -> Mux2/2
  Data Type Conversion/1 -> Display/1, Integrator/1
  Constant/1 -> Mux3/1, Mux2/1, Mux1/1, Mux/1
  Mux1/1 -> Position Blade 2/1
  Mux2/1 -> Position Blade 3/1
  Mux/1 -> Position Blade1/1
  Demux/1 -> Mux/2
  Actuators/1 -> Data Type Conversion/1
  Integrator/1 -> Gain/1
  Gain/1 -> Display1/1, Demux/1

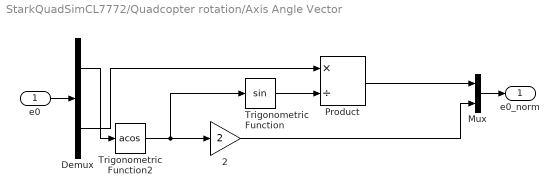
== system StarkQuadSimCL7772/Quadcopter rotation/Axis Angle Vector ==
  e0 : Inport
  2 : Gain  Gain=2  SaturateOnIntegerOverflow=on  OutDataTypeStr=Inherit: Same as input  ParamDataTypeStr=Inherit: Same as input
  Demux : Demux  Outputs=[1 3 ]
  Mux : Mux  Inputs=2
  Product : Product  Inputs=*/  SaturateOnIntegerOverflow=on  InputSameDT=on  OutDataTypeStr=Inherit: Same as first input
  Trigonometric Function : Trigonometry
  Trigonometric Function2 : Trigonometry  Operator=acos
  e0_norm : Outport
  wires:
  Demux/1 -> Trigonometric Function2/1
  Demux/2 -> Product/1
  Mux/1 -> e0_norm/1
  2/1 -> Mux/2
  Trigonometric Function2/1 -> Trigonometric Function/1, 2/1
  e0/1 -> Demux/1
  Trigonometric Function/1 -> Product/2
  Product/1 -> Mux/1

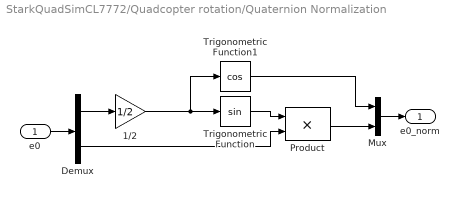
== system StarkQuadSimCL7772/Quadcopter rotation/Quaternion Normalization ==
  e0 : Inport
  1/2 : Gain  Gain=1/2  SaturateOnIntegerOverflow=on  OutDataTypeStr=Inherit: Same as input  ParamDataTypeStr=Inherit: Same as input
  Demux : Demux  Outputs=[1 3]
  Mux : Mux  Inputs=2
  Product : Product  SaturateOnIntegerOverflow=on  InputSameDT=on  OutDataTypeStr=Inherit: Same as first input
  Trigonometric Function : Trigonometry
  Trigonometric Function1 : Trigonometry  Operator=cos
  e0_norm : Outport
  wires:
  Trigonometric Function1/1 -> Mux/1
  Demux/2 -> Product/2
  Demux/1 -> 1/2/1
  Mux/1 -> e0_norm/1
  Product/1 -> Mux/2
  Trigonometric Function/1 -> Product/1
  1/2/1 -> Trigonometric Function1/1, Trigonometric Function/1
  e0/1 -> Demux/1

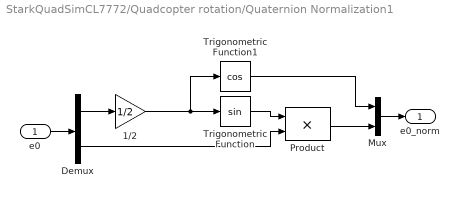
== system StarkQuadSimCL7772/Quadcopter rotation/Quaternion Normalization1 ==
  e0 : Inport
  1/2 : Gain  Gain=1/2  SaturateOnIntegerOverflow=on  OutDataTypeStr=Inherit: Same as input  ParamDataTypeStr=Inherit: Same as input
  Demux : Demux  Outputs=[1 3]
  Mux : Mux  Inputs=2
  Product : Product  SaturateOnIntegerOverflow=on  InputSameDT=on  OutDataTypeStr=Inherit: Same as first input
  Trigonometric Function : Trigonometry
  Trigonometric Function1 : Trigonometry  Operator=cos
  e0_norm : Outport
  wires:
  e0/1 -> Demux/1
  1/2/1 -> Trigonometric Function/1, Trigonometric Function1/1
  Trigonometric Function/1 -> Product/1
  Product/1 -> Mux/2
  Mux/1 -> e0_norm/1
  Demux/1 -> 1/2/1
  Demux/2 -> Product/2
  Trigonometric Function1/1 -> Mux/1

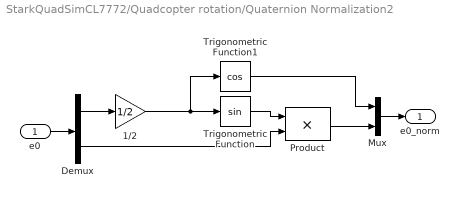
== system StarkQuadSimCL7772/Quadcopter rotation/Quaternion Normalization2 ==
  e0 : Inport
  1/2 : Gain  Gain=1/2  SaturateOnIntegerOverflow=on  OutDataTypeStr=Inherit: Same as input  ParamDataTypeStr=Inherit: Same as input
  Demux : Demux  Outputs=[1 3]
  Mux : Mux  Inputs=2
  Product : Product  SaturateOnIntegerOverflow=on  InputSameDT=on  OutDataTypeStr=Inherit: Same as first input
  Trigonometric Function : Trigonometry
  Trigonometric Function1 : Trigonometry  Operator=cos
  e0_norm : Outport
  wires:
  Trigonometric Function1/1 -> Mux/1
  Demux/2 -> Product/2
  Demux/1 -> 1/2/1
  Mux/1 -> e0_norm/1
  Product/1 -> Mux/2
  Trigonometric Function/1 -> Product/1
  1/2/1 -> Trigonometric Function1/1, Trigonometric Function/1
  e0/1 -> Demux/1
